simulink model "IMU"  (R2015a)
settings: Solver=FixedStepDiscrete  StartTime=0.0  StopTime=20  RelTol=1e-3
settings Model: SimulationMode=external  ExtModeTrigDuration=2  Creator=Francescodario  LastModifiedBy=Francescodario
settings OptimizationCC: OptimizeModelRefInitCode=on  LifeSpan=1
settings DebuggingCC: UnderspecifiedInitializationDetection=Classic  MergeDetectMultiDrivingBlocksExec=none
settings HardwareCC: ProdBitPerInt=16  ProdBitPerPointer=8  ProdIntDivRoundTo=Zero  ProdEndianess=LittleEndian  ProdWordSize=8  ProdHWDeviceType=Atmel->AVR
settings RTWCC: SystemTargetFile=realtime.tlc  GenerateMakefile=off  TemplateMakefile=realtime.tmf  Description=Run on Target Hardware  RTWVerbose=off
settings ERTTargetCC: CombineOutputUpdateFcns=off  ExtModeTransport=3  ExtModeMexFile=ext_serial_win32_comm_rtt  ExtModeMexArgs=0 1 9600  ERTSrcFileBannerTemplate=realtime_code_template.cgt  ERTHdrFileBannerTemplate=realtime_code_template.cgt  ERTDataSrcFileTemplate=realtime_code_template.cgt  ERTDataHdrFileTemplate=realtime_code_template.cgt  ERTCustomFileTemplate=realtime_file_process.tlc

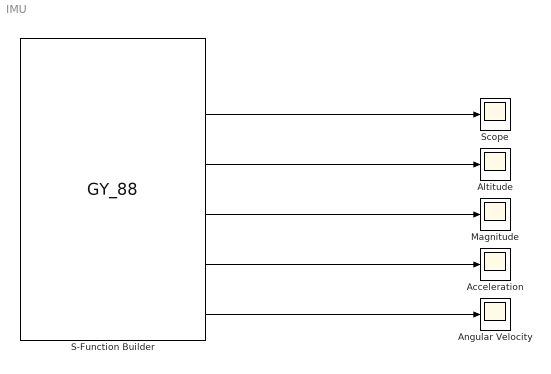
== system IMU ==
  Acceleration : Scope
      settings: SaveName=ScopeData3
  Altitude : Scope
  "Angular Velocity " : Scope
      settings: SaveName=ScopeData4
  "Magnitude " : Scope
      settings: SaveName=ScopeData2
  S-Function Builder : S-Function  InitFcn=try, set_param(gcb,'FunctionName','GY_88'), end  FunctionName=GY_88  SFunctionModules=GY_88_wrapper  mask(S-Function Builder){}
      mask help: Simulink:masks:SFunctionBuilder_MD
      mask init:
      | val = [[.9  0.75 0.75 1 1 .9 .9 1]',[1 1 0.75 0.75 .9 .9 1 .9]'];try , sys = get_param(gcb,'SfunBuilderFcnName');if isempty(sys), sys = get_param(gcb,'FunctionName'); end,catch, sys = get_param(gcb,'FunctionName'); end
      settings: CopyFcn=set_param(gcbh,'LinkStatus','none')  PreSaveFcn=try, set_param(gcb,'FunctionName','GY_88'), end  OpenFcn=sfunctionwizard(gcbh)
      mask Display: plot(val(:,1),val(:,2)),disp(sys), port_label('output',1,'temperature'), port_label('output',2,'pressure'), port_label('output',3,'altitude'), port_label('output',4,'magnitude'), port_label('output',5,'acceleration'), port_label('output',6,'angular_velocity')
  Scope : Scope
  wires:
  S-Function Builder/2 -> Scope/1
  S-Function Builder/3 -> Altitude/1
  S-Function Builder/4 -> "Magnitude "/1
  S-Function Builder/5 -> Acceleration/1
  S-Function Builder/6 -> "Angular Velocity "/1
